simulink model "frontal"  (R2020b)
settings: Solver=VariableStepAuto  StartTime=0.0  StopTime=2  RelTol=1e-3
values from neighbouring files (symbols this model uses):
  xr = -1    [avaliarFollowline.m]
undefined symbols (not defined in the file or in its folder): Kx, x0
settings Model: Creator=mmaximo  LastModifiedBy=kenji

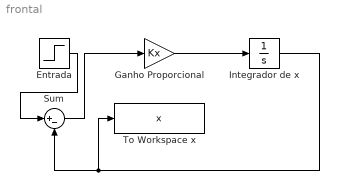
== system frontal ==
  Entrada : Step  Time=0  Before=x0  After=xr  SampleTime=0
  Ganho Proporcional : Gain  Gain=Kx
  Integrador de x : Integrator
  Sum : Sum  Inputs=|+-
  To Workspace x : ToWorkspace  VariableName=x  SaveFormat=Structure With Time  SampleTime=-1
  wires:
  Ganho Proporcional/1 -> Integrador de x/1
  Integrador de x/1 -> To Workspace x/1, Sum/2
  Sum/1 -> Ganho Proporcional/1
  Entrada/1 -> Sum/1
